simulink model "Task_3_os_academy"  (R2021a)
settings: Solver=ode1  StartTime=0.0  StopTime=5  RelTol=1e-3
libraries: simulink x3
settings Model: Creator=SA  LastModifiedBy=SA
settings OptimizationCC: DefaultParameterBehavior=Inlined  UseDivisionForNetSlopeComputation=on  GainParamInheritBuiltInType=on  UseFloatMulNetSlope=on  InlineInvariantSignals=on  PassReuseOutputArgsAs=Individual arguments  ZeroExternalMemoryAtStartup=off  ZeroInternalMemoryAtStartup=off  NoFixptDivByZeroProtection=on  EfficientFloat2IntCast=on  LifeSpan=1  OptimizeBlockOrder=speed  DifferentSizesBufferReuse=on  EfficientTunableParamExpr=on
settings DebuggingCC: ParameterTunabilityLossMsg=error
settings HardwareCC: ProdBitPerInt=16  ProdBitPerPointer=16  ProdBitPerSizeT=16  ProdBitPerPtrDiffT=16  ProdLargestAtomicFloat=None  ProdWordSize=8  ProdLongLongMode=on  ProdHWDeviceType=Atmel->AVR
settings SFSimCC: MATLABDynamicMemAlloc=off
settings RTWCC: SystemTargetFile=ert.tlc  TemplateMakefile=ert_default_tmf  PortableWordSizes=on
settings CodeAppCC: ForceParamTrailComments=on  IgnoreCustomStorageClasses=off  OperatorAnnotations=on  SimulinkDataObjDesc=on  SFDataObjDesc=on  CustomSymbolStrGlobalVar=rt$N$M  CustomSymbolStrType=$N$M  CustomSymbolStrFcn=$N$M$F  CustomSymbolStrMacro=$N$M  InsertBlockDesc=on
settings ERTTargetCC: TargetLangStandard=C99 (ISO)  GenerateSampleERTMain=on  IncludeMdlTerminateFcn=off  CombineSignalStateStructs=on  SupportComplex=off  SupportContinuousTime=on  InlinedParameterPlacement=NonHierarchical  ERTCustomFileTemplate=example_file_process.tlc  ERTFilePackagingFormat=CompactWithDataFile

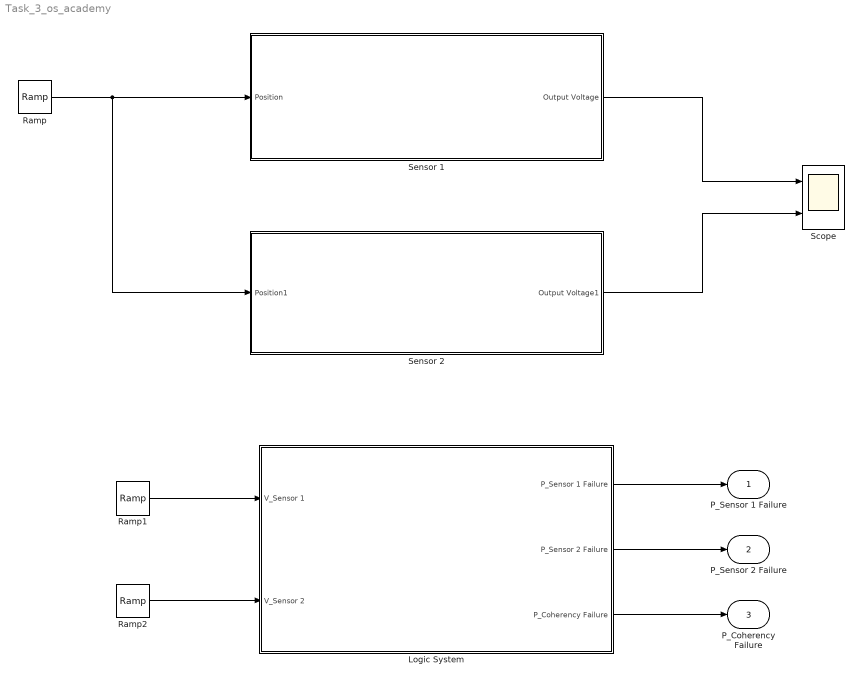
== system Task_3_os_academy ==
  Logic System : Subsystem  TreatAsAtomicUnit=on
      settings: RTWSystemCode=Nonreusable function
  Ramp : simulink/Sources/Ramp  slope=1  start=0  InitialOutput=0
  Ramp1 : simulink/Sources/Ramp  slope=1  start=0  InitialOutput=0
  Ramp2 : simulink/Sources/Ramp  slope=-1  start=0  InitialOutput=0
  Scope : Scope  NumInputPorts=2
  Sensor 1 : Subsystem
  Sensor 2 : Subsystem
  P_Sensor 1 Failure : Outport
  P_Sensor 2 Failure : Outport  Port=2
  P_Coherency Failure : Outport  Port=3
  wires:
  Sensor 1/1(Output Voltage) -> Scope/1
  Sensor 2/1(Output Voltage1) -> Scope/2
  Ramp2/1 -> Logic System/2(V_Sensor 2)
  Ramp1/1 -> Logic System/1(V_Sensor 1)
  Logic System/3(P_Coherency Failure) -> P_Coherency Failure/1
  Logic System/2(P_Sensor 2 Failure) -> P_Sensor 2 Failure/1
  Logic System/1(P_Sensor 1 Failure) -> P_Sensor 1 Failure/1
  Ramp/1 -> Sensor 2/1(Position1), Sensor 1/1(Position)

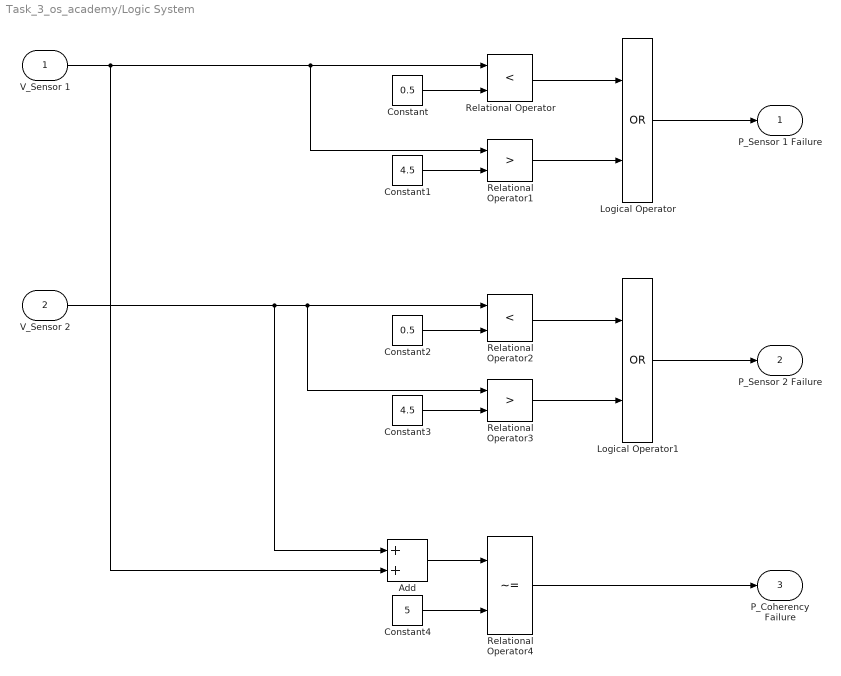
== system Task_3_os_academy/Logic System ==
  V_Sensor 1 : Inport
  V_Sensor 2 : Inport  Port=2
  Add : Sum
  Constant : Constant  Value=0.5
  Constant1 : Constant  Value=4.5
  Constant2 : Constant  Value=0.5
  Constant3 : Constant  Value=4.5
  Constant4 : Constant  Value=5
  Logical Operator : Logic  Operator=OR  AllPortsSameDT=off  OutDataTypeStr=boolean
  Logical Operator1 : Logic  Operator=OR  AllPortsSameDT=off  OutDataTypeStr=boolean
  Relational Operator : RelationalOperator  Operator=<  OutDataTypeStr=boolean  RndMeth=Simplest
  Relational Operator1 : RelationalOperator  Operator=>  OutDataTypeStr=boolean  RndMeth=Simplest
  Relational Operator2 : RelationalOperator  Operator=<  OutDataTypeStr=boolean  RndMeth=Simplest
  Relational Operator3 : RelationalOperator  Operator=>  OutDataTypeStr=boolean  RndMeth=Simplest
  Relational Operator4 : RelationalOperator  Operator=~=  OutDataTypeStr=boolean  RndMeth=Simplest
  P_Sensor 1 Failure : Outport
  P_Sensor 2 Failure : Outport  Port=2
  P_Coherency Failure : Outport  Port=3
  wires:
  Logical Operator1/1 -> P_Sensor 2 Failure/1
  Relational Operator4/1 -> P_Coherency Failure/1
  Constant4/1 -> Relational Operator4/2
  V_Sensor 2/1 -> Add/1, Relational Operator3/1, Relational Operator2/1
  Constant3/1 -> Relational Operator3/2
  Relational Operator/1 -> Logical Operator/1
  Relational Operator3/1 -> Logical Operator1/2
  Relational Operator1/1 -> Logical Operator/2
  Relational Operator2/1 -> Logical Operator1/1
  Constant2/1 -> Relational Operator2/2
  Add/1 -> Relational Operator4/1
  Logical Operator/1 -> P_Sensor 1 Failure/1
  Constant1/1 -> Relational Operator1/2
  V_Sensor 1/1 -> Add/2, Relational Operator1/1, Relational Operator/1
  Constant/1 -> Relational Operator/2

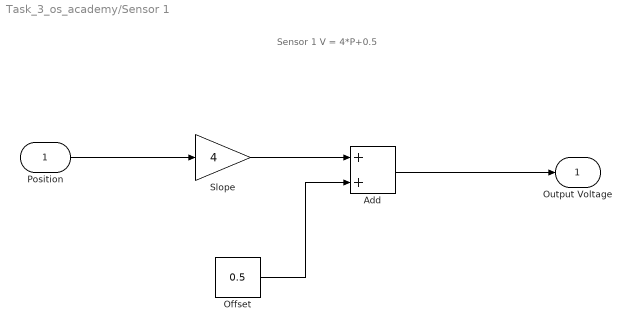
== system Task_3_os_academy/Sensor 1 ==
  note: Sensor 1
      |
      | V = 4*P+0.5
  Position : Inport
  Add : Sum
  Offset : Constant  Value=0.5
  Slope : Gain  Gain=4
  Output Voltage : Outport
  wires:
  Position/1 -> Slope/1
  Offset/1 -> Add/2
  Slope/1 -> Add/1
  Add/1 -> Output Voltage/1

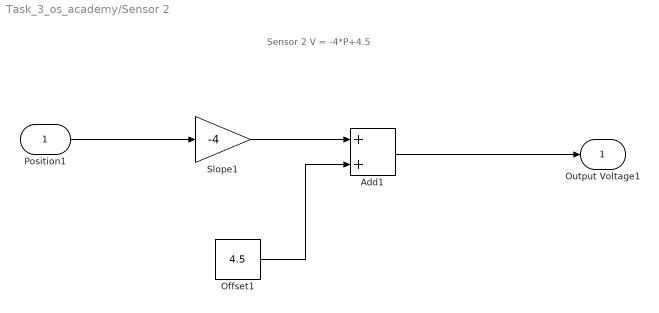
== system Task_3_os_academy/Sensor 2 ==
  note: Sensor 2
      |
      | V = -4*P+4.5
  Position1 : Inport
  Add1 : Sum
  Offset1 : Constant  Value=4.5
  Slope1 : Gain  Gain=-4
  Output Voltage1 : Outport
  wires:
  Add1/1 -> Output Voltage1/1
  Offset1/1 -> Add1/2
  Slope1/1 -> Add1/1
  Position1/1 -> Slope1/1
